simulink model "helicopter_MPC"  (R2021b)
settings: Solver=ode45  StartTime=0.0  StopTime=T  RelTol=1e-3
InitFcn:
  | hwinit
values from neighbouring files (symbols this model uses):
  A_lin = [0, 1, 0; K1*cos(alpha_ref), -b, -2*K3*omega_ref; 0, 0, -K4 ]    [observer.m]
  B_lin = [0;0; -K4]    [observer.m]
  C = [1, 0, 0; 0, 0, 1]    [MPC_step.m]    (also in contoller_4dim.m; observer.m)
  h = 0.01    [contoller_4dim.m]    (also in observer_check_EKF.m)
  N = 5    [MPC_step.m]
  Q_MPC = [5000, 0, 0; 0, 20, 0; 0, 0, 0.1]    [MPC_step.m]
  R_MPC = [80]    [MPC_step.m]
  rho = 1000    [MPC_step.m]
  u_lb = [-1]    [MPC_step.m]
  u_ub = [1]    [MPC_step.m]
  x_max = [ pi/4;  1000; 337]    [MPC_step.m]
  x_min = [-pi/4; -1000; -335]    [MPC_step.m]
  x_ref = [alpha_ref; alpha_dot_ref; omega_ref;-1]    [contoller_4dim.m]
undefined symbols (not defined in the file or in its folder): adingain, adinoffs, HeliMexHandle, P, t_mpc, y_ref_desired
libraries: simulink x1, sharedTrackingLibrary x1, eeGeneralControl x1, dspstat3 x1
settings Model: Creator=fkzhang  LastModifiedBy=lcaric
settings SolverCC: AlgebraicLoopSolver=TrustRegion
settings DataIOCC: LimitDataPoints=on  SaveFormat=Array  ReturnWorkspaceOutputs=off
settings OptimizationCC: BlockReduction=off  BooleanDataType=off  LifeSpan=inf
settings DebuggingCC: SaveWithParameterizedLinksMsg=none  UnderspecifiedInitializationDetection=Classic  MergeDetectMultiDrivingBlocksExec=none  SignalResolutionControl=TryResolveAllWithWarning  AllowSymbolicDim=off  SFUnexpectedBacktrackingDiag=warning  SFNoUnconditionalDefaultTransitionDiag=warning  SFExecutionAtInitializationDiag=none  SFMachineParentedDataDiag=warning  ArithmeticOperatorsInVariantConditions=warning
settings HardwareCC: ProdBitPerPointer=32  ProdBitPerSizeT=32  ProdBitPerPtrDiffT=32  ProdLargestAtomicFloat=None  ProdIntDivRoundTo=Undefined  ProdEndianess=Unspecified  ProdWordSize=32  ProdHWDeviceType=32-bit Generic  TargetBitPerPointer=64  TargetBitPerSizeT=64  TargetBitPerPtrDiffT=64  TargetLongLongMode=on  TargetIntDivRoundTo=Zero  TargetEndianess=LittleEndian  TargetWordSize=64  TargetHWDeviceType=MATLAB Host  ProdEqTarget=off
settings ModelReferenceCC: PropagateSignalLabelsOutOfModel=off
settings SFSimCC: SimUseLocalCustomCode=off  CustomCodeUndefinedFunction=UseInterfaceOnly
settings RTWCC: RTWUseLocalCustomCode=off
settings CodeAppCC: StateflowObjectComments=on
settings GRTTargetCC: TargetLangStandard=C89/C90 (ANSI)
settings ConfigComp: CovMetricSettings=dw  CovSaveCumulativeToWorkspaceVar=on  CovSaveSingleToWorkspaceVar=on  CovExternalEMLEnable=off  CovSFcnEnable=off

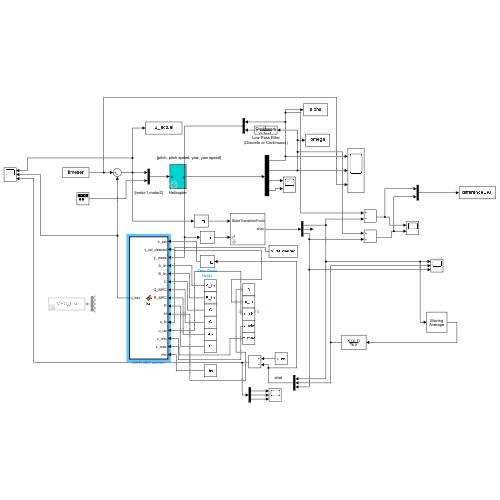
[thumbnail: Simulink's stored preview of the top-level diagram]
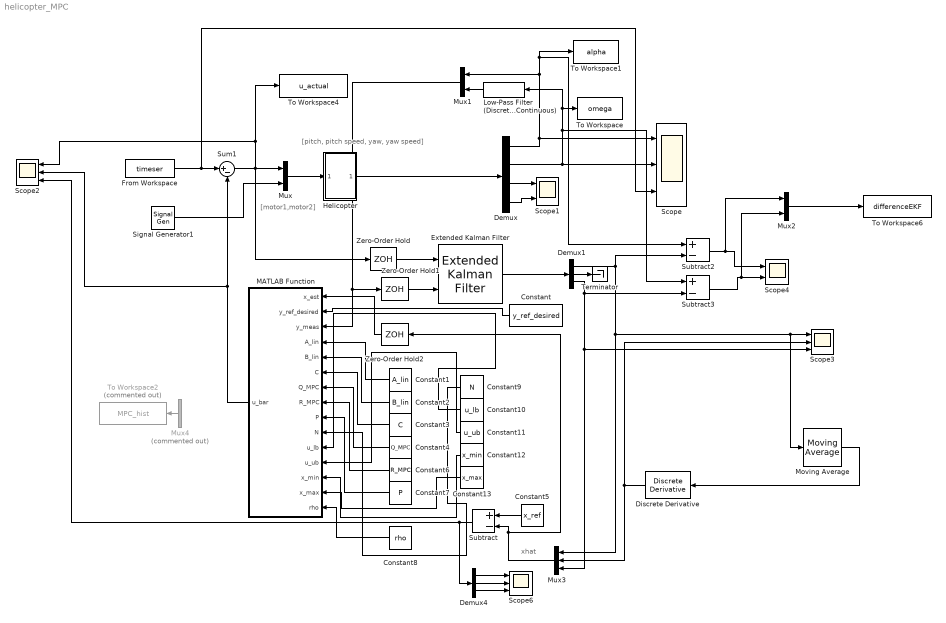
== system helicopter_MPC ==
  note: xhat
  note: [pitch, pitch speed, yaw, yaw speed]
  note: [motor1,motor2]
  Constant : Constant  Value=y_ref_desired
  Constant1 : Constant  Value=A_lin
  Constant10 : Constant  Value=u_lb
  Constant11 : Constant  Value=u_ub
  Constant12 : Constant  Value=x_min
  Constant13 : Constant  Value=x_max
  Constant2 : Constant  Value=B_lin
  Constant3 : Constant  Value=C
  Constant4 : Constant  Value=Q_MPC
  Constant5 : Constant  Value=x_ref
  Constant6 : Constant  Value=R_MPC
  Constant7 : Constant  Value=P
  Constant8 : Constant  Value=rho
  Constant9 : Constant  Value=N
  Demux : Demux
  Demux1 : Demux  Outputs=3
  Demux4 : Demux  Outputs=3
  Discrete Derivative : simulink/Discrete/Discrete Derivative  gainval=1.0  ICPrevScaledInput=0.0  OutMin=[]  OutMax=[]  OutDataType=fixdt(1, 16)  OutScaling=2^-10  DoSatur=off
  Extended Kalman Filter : sharedTrackingLibrary/Extended Kalman Filter  StateTransitionFcn=nonlin_evolution  HasStateTransitionJacobianFcn=off  StateTransitionJacobianFcn=nonlin_jacobian  HasAdditiveProcessNoise=Additive  ProcessNoise=Q_kalman  HasTimeVaryingProcessNoise=off  HasStateTransitionFcnExtraArgument=1  InitialState=[0; 0; 0]  InitialStateCovariance=Q_kalman  MeasurementFcn1=nonlin_measurement_all  HasMeasurementJacobianFcn1=off  HasMeasurementEnablePort1=off  HasAdditiveMeasurementNoise1=Additive  MeasurementNoise1=R_kalman  HasTimeVaryingMeasurementNoise1=off  HasMeasurementFcnExtraArgument1=0  MeasurementFcn2=nonlin_measurement_omega  HasMeasurementJacobianFcn2=off  HasMeasurementEnablePort2=off  HasAdditiveMeasurementNoise2=Additive  MeasurementNoise2=10  HasTimeVaryingMeasurementNoise2=off  HasMeasurementFcnExtraArgument2=0  MeasurementFcn3=myMeasurementFcn  HasMeasurementJacobianFcn3=off  HasMeasurementEnablePort3=off  HasAdditiveMeasurementNoise3=Additive  MeasurementNoise3=1  HasTimeVaryingMeasurementNoise3=off  HasMeasurementFcnExtraArgument3=0  MeasurementFcn4=myMeasurementFcn  HasMeasurementJacobianFcn4=off  HasMeasurementEnablePort4=off  HasAdditiveMeasurementNoise4=Additive  MeasurementNoise4=1  HasTimeVaryingMeasurementNoise4=off  HasMeasurementFcnExtraArgument4=0  MeasurementFcn5=myMeasurementFcn  HasMeasurementJacobianFcn5=off  HasMeasurementEnablePort5=off  HasAdditiveMeasurementNoise5=Additive  MeasurementNoise5=1  HasTimeVaryingMeasurementNoise5=off  HasMeasurementFcnExtraArgument5=0  EnableMultirate=off  StateTransitionFcnSampleTime=1  MeasurementFcn1SampleTime=1  MeasurementFcn2SampleTime=1  MeasurementFcn3SampleTime=1  MeasurementFcn4SampleTime=1  MeasurementFcn5SampleTime=1  UseCurrentEstimator=on  OutputStateCovariance=off  DataType=double  SampleTime=0.02  NumberOfMeasurements=1
      settings: SourceProductBaseCode=AE,PW,CT,DR,TF,ID,LP,NV,AR,RO,RR,UV,VE
  From Workspace : FromWorkspace  VariableName=timeser
  Helicopter : Subsystem  mask{Ts=h}
      mask prompts: Ts "sampletime"
      mask init:
      | sf_heli_init
      mask Display:
      | port_label('input',1,'u');
      | port_label('output',1,'y');
  Low-Pass Filter (Discrete or Continuous) : eeGeneralControl/Low-Pass Filter (Discrete or Continuous)  K=1  T=0.1  B=inf  A=-inf  init_option=Inherited from block input  x0=0  Ts=0
  MATLAB Function : MATLAB Function  TreatAsAtomicUnit=on
  Moving Average : dspstat3/Moving Average  Method=Sliding window  ForgettingFactorPort=off  SpecifyWindowLength=on  WindowLength=5  ForgettingFactor=0.9  SimulateUsing=Code generation
  Mux : Mux  Inputs=2
  Mux1 : Mux  Inputs=2
  Mux2 : Mux  Inputs=2
  Mux3 : Mux  Inputs=3
  Mux4 : Mux  Commented=on
  Scope{,2..3,6} (4 alike) : Scope  NumInputPorts=3
  Scope1 : Scope  NumInputPorts=2
  Scope4 : Scope  NumInputPorts=2
  Signal Generator1 : SignalGenerator  WaveForm=square  Amplitude=0  Frequency=1/20
  Subtract : Sum  Inputs=+-
  Subtract2 : Sum  Inputs=+-
  Subtract3 : Sum  Inputs=+-
  Sum1 : Sum  Inputs=|+-
  Terminator : Terminator
  To Workspace : ToWorkspace  VariableName=omega  SaveFormat=Timeseries  SampleTime=-1
  To Workspace1 : ToWorkspace  VariableName=alpha  SaveFormat=Timeseries  SampleTime=-1
  To Workspace2 : ToWorkspace  Commented=on  VariableName=MPC_hist  SaveFormat=Timeseries  SampleTime=-1
  To Workspace4 : ToWorkspace  VariableName=u_actual  SaveFormat=Timeseries  SampleTime=-1
  To Workspace6 : ToWorkspace  VariableName=differenceEKF  SaveFormat=Timeseries  SampleTime=-1
  Zero-Order Hold : ZeroOrderHold  SampleTime=0.02
  Zero-Order Hold1 : ZeroOrderHold  SampleTime=0.02
  Zero-Order Hold2 : ZeroOrderHold  SampleTime=t_mpc
  wires:
  Mux/1 -> Helicopter/1(In1)
  Signal Generator1/1 -> Mux/2
  Demux/2 -> Low-Pass Filter (Discrete or Continuous)/1, To Workspace/1, Subtract3/1, Scope/2
  Demux/3 -> Scope1/1
  Demux/4 -> Scope1/2
  From Workspace/1 -> Sum1/1, Scope/3
  Demux/1 -> Subtract2/1, To Workspace1/1, Mux1/1, Scope/1
  Mux1/1 -> MATLAB Function/3(y_meas), Zero-Order Hold1/1
  Helicopter/1(Out1) -> Demux/1
  Sum1/1 -> To Workspace4/1, Scope2/1, Zero-Order Hold/1, Mux/1
  Subtract/1 -> Scope2/3, Demux4/1
  Constant5/1 -> Subtract/1
  Zero-Order Hold/1 -> Extended Kalman Filter/1
  Zero-Order Hold1/1 -> Extended Kalman Filter/2
  Extended Kalman Filter/1 -> Demux1/1
  Demux1/3 -> Subtract3/2, Mux3/3, Scope3/3
  Subtract2/1 -> Mux2/1, Scope4/1
  Subtract3/1 -> Mux2/2, Scope4/2
  Mux2/1 -> To Workspace6/1
  Low-Pass Filter (Discrete or Continuous)/1 -> Mux1/2
  Demux1/1 -> Subtract2/2, Mux3/1, Moving Average/1, Scope3/1
  Discrete Derivative/1 -> Scope3/2, Mux3/2
  Mux3/1 -> Subtract/2, Zero-Order Hold2/1
  Moving Average/1 -> Discrete Derivative/1
  Demux1/2 -> Terminator/1
  Demux4/1 -> Scope6/1
  Demux4/3 -> Scope6/3
  Demux4/2 -> Scope6/2
  MATLAB Function/1(u_bar) -> Scope2/2, Sum1/2
  Constant/1 -> MATLAB Function/2(y_ref_desired)
  Mux4/1 -> To Workspace2/1
  Zero-Order Hold2/1 -> MATLAB Function/1(x_est)
  Constant1/1 -> MATLAB Function/4(A_lin)
  Constant2/1 -> MATLAB Function/5(B_lin)
  Constant3/1 -> MATLAB Function/6(C)
  Constant4/1 -> MATLAB Function/7(Q_MPC)
  Constant6/1 -> MATLAB Function/8(R_MPC)
  Constant7/1 -> MATLAB Function/9(P)
  Constant9/1 -> MATLAB Function/10(N)
  Constant10/1 -> MATLAB Function/11(u_lb)
  Constant11/1 -> MATLAB Function/12(u_ub)
  Constant12/1 -> MATLAB Function/13(x_min)
  Constant13/1 -> MATLAB Function/14(x_max)
  Constant8/1 -> MATLAB Function/15(rho)

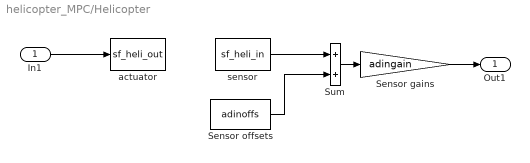
== system helicopter_MPC/Helicopter ==
  In1 : Inport
  Sensor gains : Gain  Gain=adingain
  Sensor offsets : Constant  Value=adinoffs
  Sum : Sum
  actuator : M-S-Function  FunctionName=sf_heli_out  Parameters=HeliMexHandle,Ts
  sensor : M-S-Function  FunctionName=sf_heli_in  Parameters=HeliMexHandle
  Out1 : Outport  VectorParamsAs1DForOutWhenUnconnected=off
  wires:
  sensor/1 -> Sum/1
  In1/1 -> actuator/1
  Sensor offsets/1 -> Sum/2
  Sum/1 -> Sensor gains/1
  Sensor gains/1 -> Out1/1

== matlab function helicopter_MPC/MATLAB Function ==
  data: x_est input; u_bar output; y_ref_desired input; y_meas input; A_lin input; B_lin input; C input; Q_MPC input; R_MPC input; P input; N input; u_lb input; u_ub input; x_min input; x_max input; rho input
function u_bar  = fcn(x_est, y_ref_desired, y_meas, A_lin, B_lin, C, Q_MPC, R_MPC, P, N, u_lb, u_ub, x_min, x_max, rho)

    u_bar = MPC_step(x_est, y_ref_desired, y_meas, A_lin, B_lin, C, Q_MPC, R_MPC, P, N, u_lb, u_ub, x_min, x_max, rho);
%     x_hist = zeros(N_sim+1, n_x); x_hist(1,:) = x0';
%     y_hist = zeros(N_sim+1, n_y);
%     u_hist = zeros(N_sim, n_u);
%     d_err = zeros(N_sim+1, 1);
%     hist_arr(3,t,:) = u_bar(1,:);
%     hist_arr(1,t+1,:) = (A_d * x_hist(t,:)' + B_d * u_hist(t,:)')';
%     hist_arr(2,t+1,:) = (C * x_hist(t+1,:)' + d_true)';
%     hist_arr(4,t) = norm(d_hat);

end
